simulink model "subjectVehicle"  (Simulink 7.5)
settings: Solver=ode3  SolverMode=SingleTasking  StartTime=0.0  StopTime=10.0  FixedStep=0.005  RelTol=1e-3
undefined symbols (not defined in the file or in its folder): detectionRange, driverReacionTime, frictionCoef, subjectPosition, subjectVelocity
settings Model: Creator=Josef  LastModifiedBy=Josef
settings OptimizationCC: BlockReduction=off  BooleanDataType=off  ExpressionDepthLimit=128
settings DebuggingCC: SaveWithParameterizedLinksMsg=none  UnderspecifiedInitializationDetection=Simplified  MergeDetectMultiDrivingBlocksExec=error  SignalResolutionControl=TryResolveAllWithWarning  SolverPrmCheckMsg=none  FcnCallInpInsideContextMsg=Enable All  StateNameClashWarn=none
settings HardwareCC: ProdIntDivRoundTo=Zero  ProdEndianess=LittleEndian  ProdHWDeviceType=Intel->x86-32 (Windows32)  TargetUnknown=on
settings ModelReferenceCC: ModelReferenceMinAlgLoopOccurrences=on
settings CodeAppCC: CustomSymbolStrType=$N$R$M_T
settings GRTTargetCC: TargetFunctionLibrary=C89/C90 (ANSI)

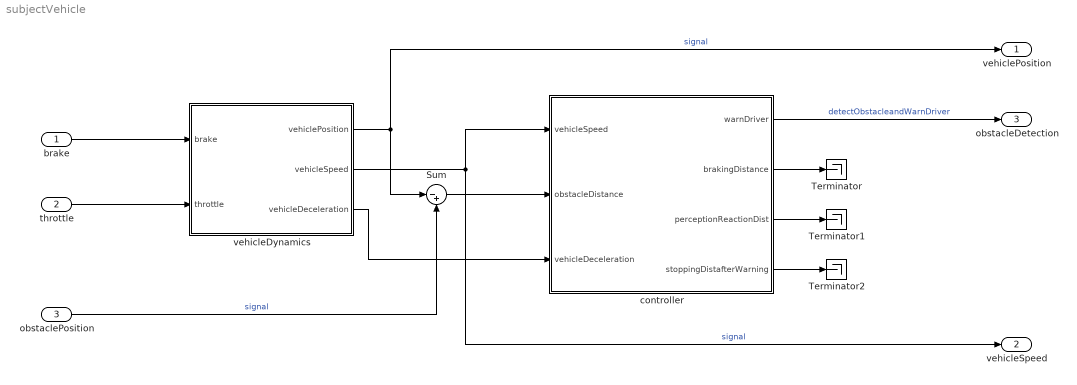
== system subjectVehicle ==
  brake : Inport
  throttle : Inport  Port=2
  obstaclePosition : Inport  Port=3
      settings: AttributesFormatString=signal
  Sum : Sum  Inputs=|-+
  Terminator : Terminator
  Terminator1 : Terminator
  Terminator2 : Terminator
  controller : Subsystem
      settings: AttributesFormatString=CWS
  vehicleDynamics : Subsystem
  vehiclePosition : Outport
      settings: AttributesFormatString=signal
  vehicleSpeed : Outport  Port=2
      settings: AttributesFormatString=signal
  obstacleDetection : Outport  Port=3
      settings: AttributesFormatString=signal
  wires:
  vehicleDynamics/1(vehiclePosition) -> Sum/1, vehiclePosition/1  "signal"
  vehicleDynamics/2(vehicleSpeed) -> controller/1(vehicleSpeed), vehicleSpeed/1  "signal"
  controller/1(warnDriver) -> obstacleDetection/1  "detectObstacleandWarnDriver"
  throttle/1 -> vehicleDynamics/2(throttle)
  brake/1 -> vehicleDynamics/1(brake)
  Sum/1 -> controller/2(obstacleDistance)
  obstaclePosition/1 -> Sum/2  "signal"
  controller/2(brakingDistance) -> Terminator/1
  vehicleDynamics/3(vehicleDeceleration) -> controller/3(vehicleDeceleration)
  controller/3(perceptionReactionDist) -> Terminator1/1
  controller/4(stoppingDistafterWarning) -> Terminator2/1

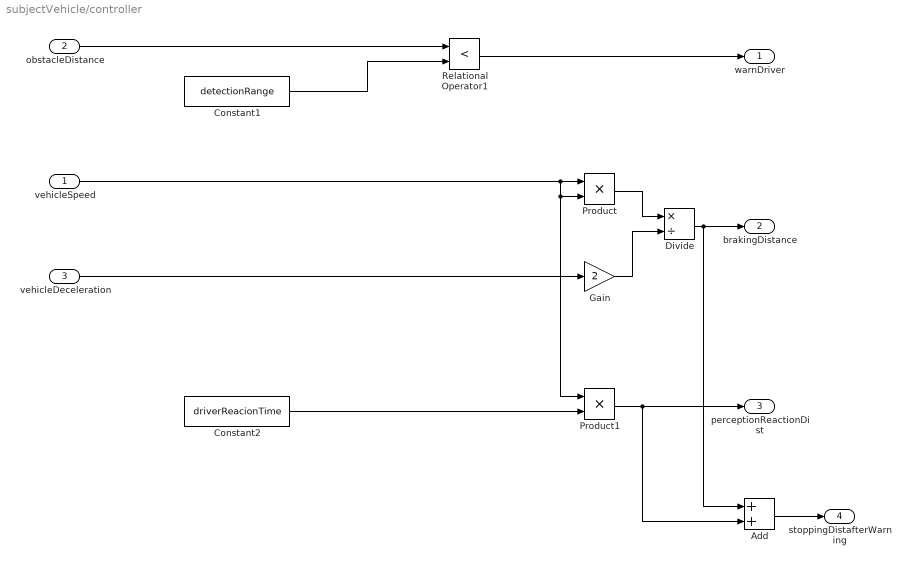
== system subjectVehicle/controller ==
  vehicleSpeed : Inport
      settings: AttributesFormatString=signal
  obstacleDistance : Inport  Port=2
      settings: AttributesFormatString=signal
  vehicleDeceleration : Inport  Port=3
      settings: AttributesFormatString=signal
  Add : Sum
  Constant1 : Constant  Value=detectionRange
  Constant2 : Constant  Value=driverReacionTime
  Divide : Product  Inputs=*/
  Gain : Gain  Gain=2
  Product : Product
  Product1 : Product
  Relational Operator1 : RelationalOperator  Operator=<  OutDataTypeStr=boolean  LogicOutDataTypeMode=boolean
  warnDriver : Outport
      settings: AttributesFormatString=detectObstacleandWarnDriver
  brakingDistance : Outport  Port=2
  perceptionReactionDist : Outport  Port=3
  stoppingDistafterWarning : Outport  Port=4
  wires:
  obstacleDistance/1 -> Relational Operator1/1
  Relational Operator1/1 -> warnDriver/1
  vehicleDeceleration/1 -> Gain/1
  Gain/1 -> Divide/2
  Product/1 -> Divide/1
  vehicleSpeed/1 -> Product/1, Product/2, Product1/1
  Divide/1 -> Add/1, brakingDistance/1
  Product1/1 -> Add/2, perceptionReactionDist/1
  Constant2/1 -> Product1/2
  Add/1 -> stoppingDistafterWarning/1
  Constant1/1 -> Relational Operator1/2

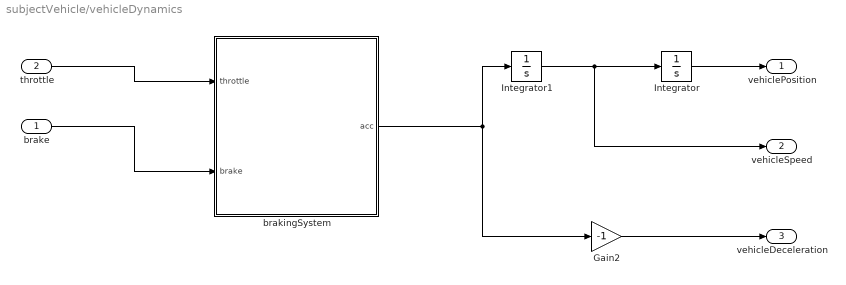
== system subjectVehicle/vehicleDynamics ==
  brake : Inport
  throttle : Inport  Port=2
  Gain2 : Gain  Gain=-1
  Integrator : Integrator  InitialCondition=subjectPosition
  Integrator1 : Integrator  InitialCondition=subjectVelocity  LimitOutput=on  LowerSaturationLimit=0
  brakingSystem : Subsystem
  vehiclePosition : Outport
      settings: AttributesFormatString=signal
  vehicleSpeed : Outport  Port=2
      settings: AttributesFormatString=signal
  vehicleDeceleration : Outport  Port=3
      settings: AttributesFormatString=signal
  wires:
  Integrator/1 -> vehiclePosition/1
  Integrator1/1 -> vehicleSpeed/1, Integrator/1
  Gain2/1 -> vehicleDeceleration/1
  brakingSystem/1(acc) -> Integrator1/1, Gain2/1
  throttle/1 -> brakingSystem/1(throttle)
  brake/1 -> brakingSystem/2(brake)

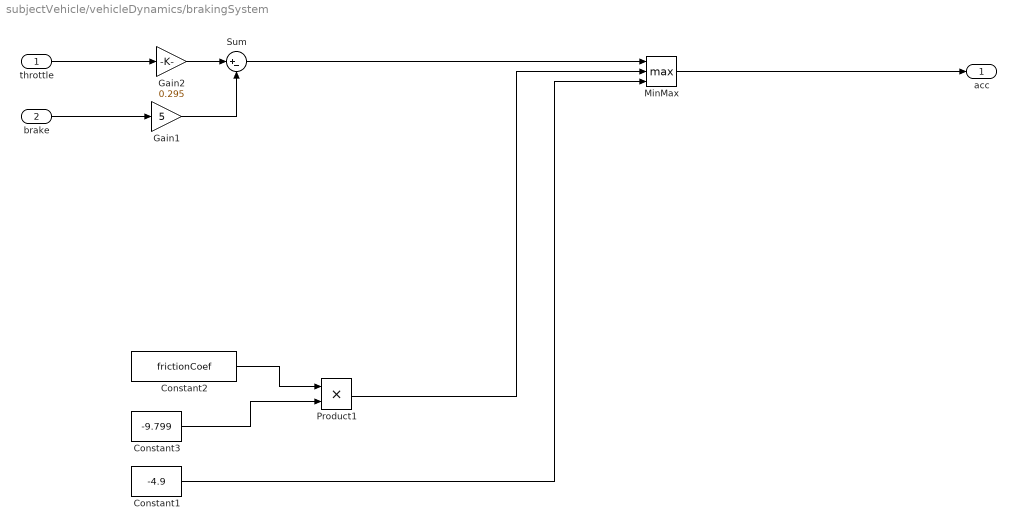
== system subjectVehicle/vehicleDynamics/brakingSystem ==
  throttle : Inport
  brake : Inport  Port=2
  Constant1 : Constant  Value=-4.9
  Constant2 : Constant  Value=frictionCoef
  Constant3 : Constant  Value=-9.799
  Gain1 : Gain  Gain=5
  Gain2 : Gain  Gain=0.295
  MinMax : MinMax  Function=max  Inputs=3
  Product1 : Product
  Sum : Sum  Inputs=|+-
  acc : Outport
  wires:
  throttle/1 -> Gain2/1
  brake/1 -> Gain1/1
  Product1/1 -> MinMax/2
  Constant1/1 -> MinMax/3
  Constant2/1 -> Product1/1
  Constant3/1 -> Product1/2
  Sum/1 -> MinMax/1
  MinMax/1 -> acc/1
  Gain1/1 -> Sum/2
  Gain2/1 -> Sum/1
